simulink model "interpolador"  (R2012b)
settings: Solver=ode3  StartTime=0.0  StopTime=10.0  FixedStep=1e-4  RelTol=1e-3
undefined symbols (not defined in the file): A, B, C
libraries: simulink x2, Encoder x2
settings Model: Creator=h3now  LastModifiedBy=h3now

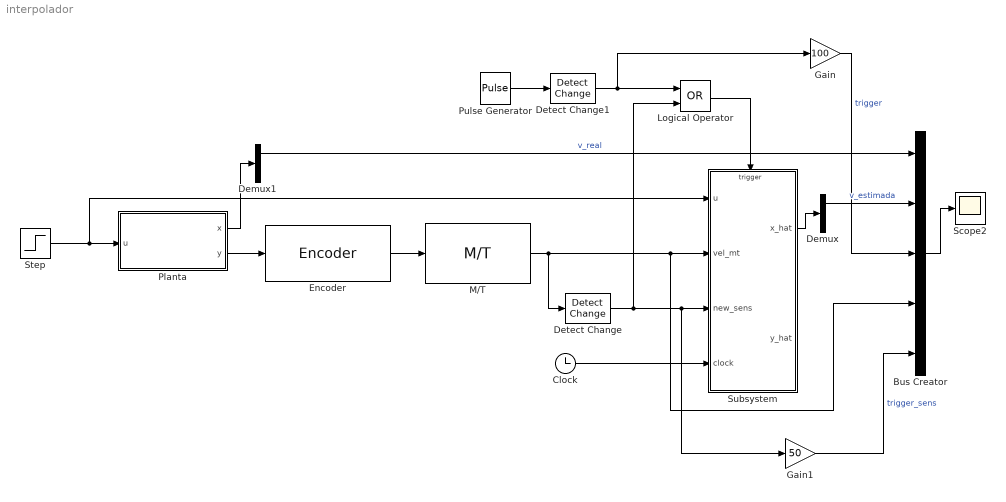
== system interpolador ==
  Bus Creator : BusCreator  Inputs=5
  Clock : Clock
  Demux : Demux  Outputs=2
  Demux1 : Demux  Outputs=2
  Detect Change : simulink/Logic and Bit Operations/Detect Change  vinit=0  InputProcessing=Inherited  OutDataTypeStr=boolean
  Detect Change1 : simulink/Logic and Bit Operations/Detect Change  vinit=0  InputProcessing=Inherited  OutDataTypeStr=boolean
  Encoder : Encoder/Encoder  Nr=10
  Gain : Gain  Gain=100  OutDataTypeStr=double
  Gain1 : Gain  Gain=50  OutDataTypeStr=double
  Logical Operator : Logic  Operator=OR  AllPortsSameDT=off  OutDataTypeStr=boolean
  M/T : Encoder/M//T  Ts=0.1
  Planta : Subsystem
  Pulse Generator : DiscretePulseGenerator  PulseType=Time based  Period=0.3  PulseWidth=50
  Scope2 : Scope
      settings: ShowLegends=on  YMin=65  YMax=160  SaveName=ScopeData2
  Step : Step  Time=5  Before=5  After=-5  SampleTime=0
  Subsystem : Subsystem
  wires:
  Encoder/1 -> M/T/1
  Planta/2(y) -> Encoder/1
  M/T/1 -> Detect Change/1, Bus Creator/4, Subsystem/2(vel_mt)
  Step/1 -> Subsystem/1(u), Planta/1(u)
  Demux/1 -> Bus Creator/2  "v_estimada"
  Planta/1(x) -> Demux1/1
  Demux1/1 -> Bus Creator/1  "v_real"
  Bus Creator/1 -> Scope2/1
  Detect Change/1 -> Logical Operator/2, Gain1/1, Subsystem/3(new_sens)
  Clock/1 -> Subsystem/4(clock)
  Subsystem/1(x_hat) -> Demux/1
  Pulse Generator/1 -> Detect Change1/1
  Detect Change1/1 -> Gain/1, Logical Operator/1
  Logical Operator/1 -> Subsystem/Trigger
  Gain/1 -> Bus Creator/3  "trigger"
  Gain1/1 -> Bus Creator/5  "trigger_sens"

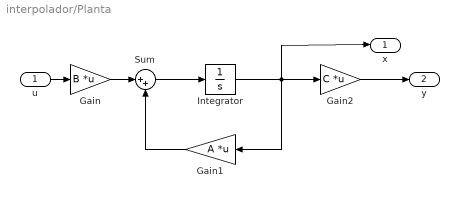
== system interpolador/Planta ==
  u : Inport
  Gain : Gain  Gain=B  Multiplication=Matrix(K*u)
  Gain1 : Gain  Gain=A  Multiplication=Matrix(K*u)
  Gain2 : Gain  Gain=C  Multiplication=Matrix(K*u)
  Integrator : Integrator
  Sum : Sum  Inputs=|++
  x : Outport
  y : Outport  Port=2
  wires:
  u/1 -> Gain/1
  Integrator/1 -> x/1, Gain2/1, Gain1/1
  Gain2/1 -> y/1
  Sum/1 -> Integrator/1
  Gain1/1 -> Sum/2
  Gain/1 -> Sum/1

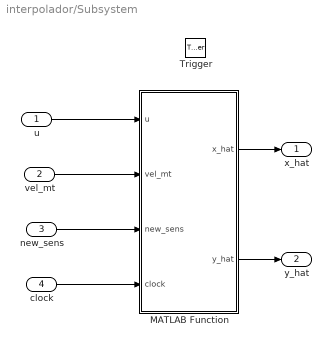
== system interpolador/Subsystem ==
  u : Inport
  vel_mt : Inport  Port=2
  new_sens : Inport  Port=3
  clock : Inport  Port=4
  Trigger : TriggerPort  PortDimensions=1
  MATLAB Function : MATLAB Function  TreatAsAtomicUnit=on
  x_hat : Outport
  y_hat : Outport  Port=2
  wires:
  new_sens/1 -> MATLAB Function/3(new_sens)
  clock/1 -> MATLAB Function/4(clock)
  vel_mt/1 -> MATLAB Function/2(vel_mt)
  u/1 -> MATLAB Function/1(u)
  MATLAB Function/1(x_hat) -> x_hat/1
  MATLAB Function/2(y_hat) -> y_hat/1

== matlab function interpolador/Subsystem/MATLAB Function ==
  data: u input; x_hat output; vel_mt input; new_sens input; clock input; y_hat output
function [x_hat,y_hat] = fcn(u, vel_mt, new_sens, clock)

    %#codegen
    persistent x;
    persistent t;
    persistent t_sens;
    persistent C;
    persistent D;

    if(isempty(x))
        x = [0 ; 0];
        t = 0;
        t_sens = t;
        C = [0 1];
        D = 0;
    end

     if(new_sens == 1)
        x = [vel_mt x(2)]';
        t_sens = clock;
     else
        deltaT = clock-max(t,t_sens);
        A = [1-0.2*deltaT 0 ; deltaT 1];
        B = [10*deltaT; 0];
        x = A*x+B*u;
        t = clock;
    end
    
    x_hat = x;
    y_hat = C*x+D*u;
end
